simulink model "synapse_plots"  (R2022a)
settings: Solver=VariableStepAuto  StartTime=0.0  StopTime=10.0  RelTol=1e-3
libraries: neuromorphic_blocks x5
settings Model: Creator=chris  LastModifiedBy=chris

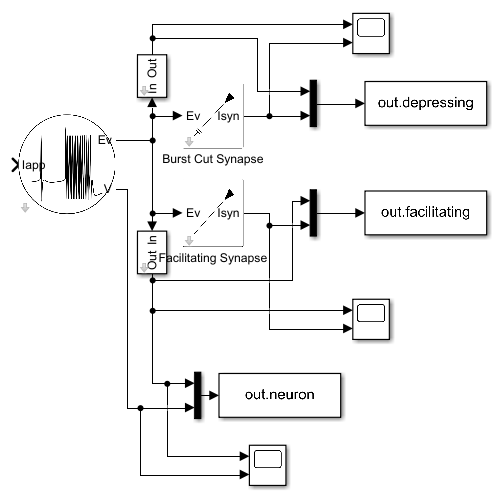
[thumbnail: Simulink's stored preview of the top-level diagram]
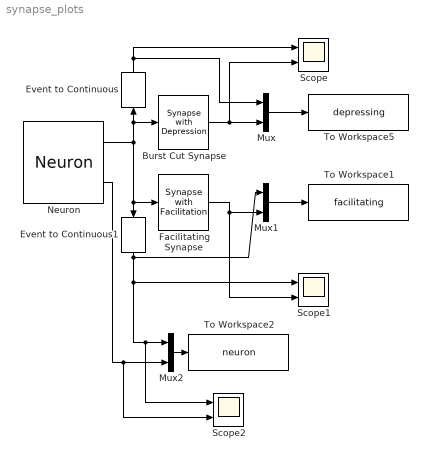
== system synapse_plots ==
  Burst Cut Synapse : neuromorphic_blocks/Neural Blocks/Synapse with Depression  gsyn_source=Internal  gsyn=2  dsyn=1.5  msyn=5  dsyn_dep=8  msyn_dep=50  timescale=0.004  rel_facilitation=sqrt(10)  rel_depression=100  input=Events  gsyn_in=0  dsyn_in=0  msyn_in=1
      settings: SourceProductName=Neuromorphic Toolbox
  Event to Continuous : neuromorphic_blocks/Events Transmission Blocks/Event to Continuous  gain=1
      settings: SourceProductName=Neuromorphic Toolbox
  Event to Continuous1 : neuromorphic_blocks/Events Transmission Blocks/Event to Continuous  gain=1
      settings: SourceProductName=Neuromorphic Toolbox
  Facilitating Synapse : neuromorphic_blocks/Neural Blocks/Synapse with Facilitation  gsyn_source=Internal  gsyn=2  dsyn=1.5  msyn=5  timescale=0.004  rel_timescale=10  input=Events  gsyn_in=0  dsyn_in=0  msyn_in=1
      settings: SourceProductName=Neuromorphic Toolbox
  Mux : Mux  Inputs=2
  Mux1 : Mux  Inputs=2
  Mux2 : Mux  Inputs=2
  Neuron : neuromorphic_blocks/Neural Blocks/Neuron  gfm_source=Internal  gfm=3  gsp_source=Internal  gsp=6  gsm_source=Internal  gsm=2  gup_source=Internal  gup=4  gum_source=Internal  gum=2  dfm=0  dsp=0.5  dsm=-0.5  dup=-0.5  dum=-1  mfm=1  msp=1  msm=1  mup=1  mum=1  timescale=0.004  rel_membrane=0.1  rel_fast=0.1  rel_slow=4  rel_ultraslow=200  Iapp_base=0.1  V0=-1.2  tresh=0  output=Both
      settings: SourceProductName=Neuromorphic Toolbox
  Scope : Scope  NumInputPorts=2
  Scope1 : Scope  NumInputPorts=2
  Scope2 : Scope  NumInputPorts=2
  To Workspace1 : ToWorkspace  VariableName=facilitating  SaveFormat=Structure With Time  SampleTime=-1
  To Workspace2 : ToWorkspace  VariableName=neuron  SaveFormat=Structure With Time  SampleTime=-1
  To Workspace5 : ToWorkspace  VariableName=depressing  SaveFormat=Structure With Time  SampleTime=-1
  wires:
  Burst Cut Synapse/1 -> Scope/2, Mux/2
  Facilitating Synapse/1 -> Mux1/2, Scope1/2
  Mux/1 -> To Workspace5/1
  Mux1/1 -> To Workspace1/1
  Neuron/1 -> Event to Continuous1/1, Facilitating Synapse/1, Burst Cut Synapse/1, Event to Continuous/1
  Event to Continuous1/1 -> Scope2/1, Mux2/1, Scope1/1, Mux1/1
  Event to Continuous/1 -> Scope/1, Mux/1
  Mux2/1 -> To Workspace2/1
  Neuron/2 -> Scope2/2, Mux2/2
